simulink model "MPC_backend_main"  (R2026a)
settings: Solver=FixedStepAuto
undefined symbols (not defined in the file or in its folder): acados_nominal_input
libraries: simulink x1
settings Model: Creator=rayyu  LastModifiedBy=rayyu
settings RTWCC: SystemTargetFile=ert.tlc  Description=Embedded Coder
settings ERTTargetCC: GenerateSampleERTMain=on

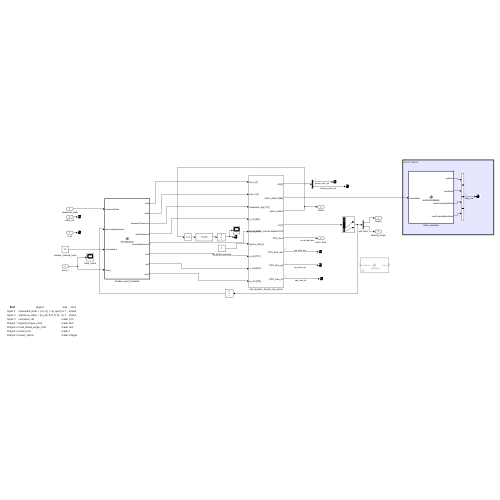
[thumbnail: Simulink's stored preview of the top-level diagram]
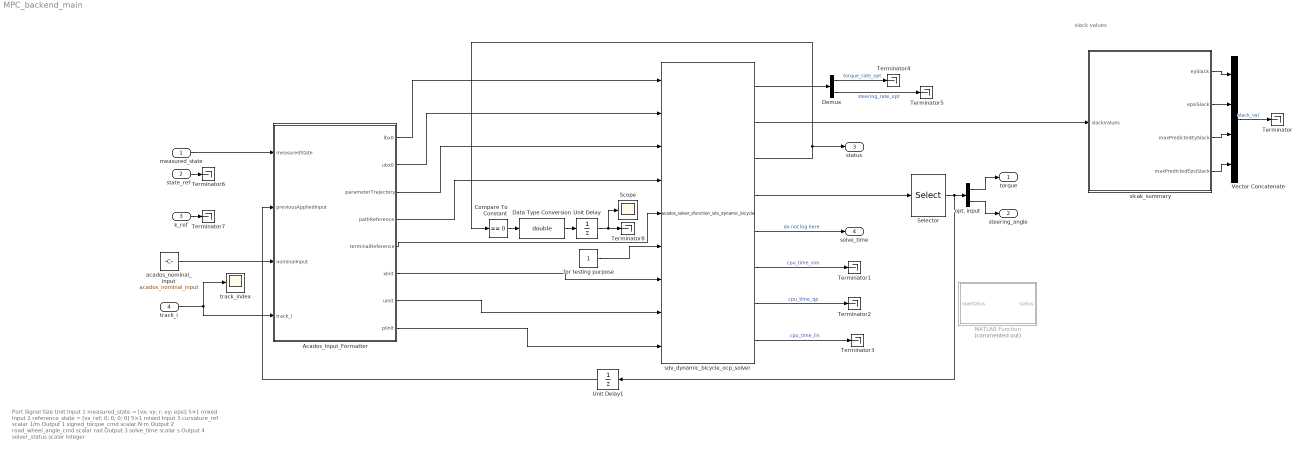
== system MPC_backend_main ==
  note: slack values
  note: Port
      | Signal
      | Size
      | Unit
      |
      | Input 1
      | measured_state = [vx; vy; r; ey; epsi]
      | 5×1
      | mixed
      |
      | Input 2
      | reference_state = [vx_ref; 0; 0; 0; 0]
      | 5×1
      | mixed
      |
      | Input 3
      | curvature_ref
      | scalar
      | 1/m
      |
      | Output 1
      | signed_torque_cmd
      | scalar
      | N·m
      |
      | Output 2
      | road_wheel_angle_cmd
      | scalar
      | rad
      |
      | Output 3
      | solve_time
      | scalar
      | s
      |
      | Output 4
      | solver_status
      | scalar
      | integer
  measured_state : Inport  PortDimensions=[5 1]
  state_ref : Inport  Port=2  PortDimensions=[1 5]
  k_ref : Inport  Port=3  PortDimensions=1
  track_i : Inport  Port=4
  Acados_Input_Formatter : MATLAB Function  TreatAsAtomicUnit=on
  Compare To Constant : simulink/Logic and Bit Operations/Compare To Constant  relop===  const=0  OutDataTypeStr=boolean
  Data Type Conversion : DataTypeConversion  OutDataTypeStr=double  SaturateOnIntegerOverflow=off  RndMeth=Floor
  Demux : Demux  Outputs=2
  MATLAB Function : MATLAB Function  Commented=on  TreatAsAtomicUnit=on
  Scope : Scope
      settings: ActiveDisplayYMinimum=-0.21951243413364641  ActiveDisplayYMaximum=1.6696874989313319
  Selector : Selector  InputPortWidth=7  IndexOptions=Index vector (dialog)  Indices=[6,7]  OutputSizes=1
  Terminator{,1..8} (9 alike) : Terminator
  Unit Delay : UnitDelay  InitialCondition=1  SampleTime=-1
  Unit Delay1 : UnitDelay  SampleTime=-1
  Vector Concatenate : Concatenate  NumInputs=4
  acados_nominal_input : Constant  Value=acados_nominal_input  VectorParams1D=off
  for testing purpose : Constant
  opt. input : Demux  Outputs=2
  sdv_dynamic_bicycle_ocp_solver : S-Function  FunctionName=acados_solver_sfunction_sdv_dynamic_bicycle  SFunctionDeploymentMode=off  EnableBusSupport=off
      mask Display:
      | port_label('input', 1, 'lbx_0 [7]')
      | port_label('input', 2, 'ubx_0 [7]')
      | port_label('input', 3, 'parameter_traj [101]')
      | port_label('input', 4, 'y_ref [891]')
      | port_label('input', 5, 'y_ref_e [5]')
      | port_label('input', 6, 'ignore_inits [1]')
      | port_label('input', 7, 'x_init [707]')
      | port_label('input', 8, 'u_init [200]')
      | port_label('input', 9, 'pi_init [700]')
      | port_label('output', 1, 'u0 [2]')
      | port_label('output', 2, 'slack_values [396]')
      | port_label('output', 3, 'solver_status')
      | port_label('output', 4, 'x1 [7]')
      | port_label('output', 5, 'CPU_time')
      | port_label('output', 6, 'CPU_time_sim')
      | port_label('output', 7, 'CPU_time_qp')
      | port_label('output', 8, 'CPU_time_lin')
      | disp('sdv_dynamic_bicycle acados OCP')
  slcak_summary : MATLAB Function  TreatAsAtomicUnit=on
  track_index : Scope
      settings: ActiveDisplayYMinimum=127.93419653260979  ActiveDisplayYMaximum=131.89125671947426
  torque : Outport
  steering_angle : Outport  Port=2
  status : Outport  Port=3
  solve_time : Outport  Port=4
  wires:
  sdv_dynamic_bicycle_ocp_solver/7 -> Terminator2/1  "cpu_time_qp"
  slcak_summary/3(maxPredictedEySlack) -> Vector Concatenate/3
  opt. input/1 -> torque/1
  Compare To Constant/1 -> Data Type Conversion/1
  Acados_Input_Formatter/5(terminalReference) -> sdv_dynamic_bicycle_ocp_solver/5
  Acados_Input_Formatter/7(uInit) -> sdv_dynamic_bicycle_ocp_solver/8
  Acados_Input_Formatter/2(ubx0) -> sdv_dynamic_bicycle_ocp_solver/2
  measured_state/1 -> Acados_Input_Formatter/1(measuredState)
  track_i/1 -> track_index/1, Acados_Input_Formatter/4(track_i)
  slcak_summary/4(maxPredictedEpsiSlack) -> Vector Concatenate/4
  sdv_dynamic_bicycle_ocp_solver/3 -> Compare To Constant/1, status/1
  sdv_dynamic_bicycle_ocp_solver/1 -> Demux/1
  sdv_dynamic_bicycle_ocp_solver/8 -> Terminator3/1  "cpu_time_lin"
  slcak_summary/2(epsiSlack) -> Vector Concatenate/2
  Vector Concatenate/1 -> Terminator/1  "slack_val"
  sdv_dynamic_bicycle_ocp_solver/5 -> solve_time/1  "do not log here"
  Acados_Input_Formatter/3(parameterTrajectory) -> sdv_dynamic_bicycle_ocp_solver/3
  sdv_dynamic_bicycle_ocp_solver/6 -> Terminator1/1  "cpu_time_sim"
  Data Type Conversion/1 -> Unit Delay/1
  Acados_Input_Formatter/1(lbx0) -> sdv_dynamic_bicycle_ocp_solver/1
  Acados_Input_Formatter/6(xInit) -> sdv_dynamic_bicycle_ocp_solver/7
  acados_nominal_input/1 -> Acados_Input_Formatter/3(nominalInput)
  Acados_Input_Formatter/8(piInit) -> sdv_dynamic_bicycle_ocp_solver/9
  slcak_summary/1(eySlack) -> Vector Concatenate/1
  Acados_Input_Formatter/4(pathReference) -> sdv_dynamic_bicycle_ocp_solver/4
  opt. input/2 -> steering_angle/1
  sdv_dynamic_bicycle_ocp_solver/4 -> Selector/1
  Unit Delay1/1 -> Acados_Input_Formatter/2(previousAppliedInput)
  Selector/1 -> Unit Delay1/1, opt. input/1
  Demux/1 -> Terminator4/1  "torque_rate_opt"
  Demux/2 -> Terminator5/1  "steering_rate_opt"
  Unit Delay/1 -> Terminator8/1, Scope/1
  state_ref/1 -> Terminator6/1
  k_ref/1 -> Terminator7/1
  for testing purpose/1 -> sdv_dynamic_bicycle_ocp_solver/6
  sdv_dynamic_bicycle_ocp_solver/2 -> slcak_summary/1(slackValues)

== matlab function MPC_backend_main/MATLAB Function ==
  data: rawStatus input; status output
function status = mapStatus(rawStatus)
if rawStatus == 0
    status = 1;
else
    status = -1;
end

end

== matlab function MPC_backend_main/Acados_Input_Formatter ==
  data: measuredState input; previousAppliedInput input; nominalInput input; track_i input; track_ref_table parameter; lbx0 output; ubx0 output; parameterTrajectory output; pathReference output; terminalReference output; xInit output; uInit output; piInit output
function [ ...
    lbx0, ...
    ubx0, ...
    parameterTrajectory, ...
    pathReference, ...
    terminalReference, ...
    xInit, ...
    uInit, ...
    piInit] = ...
    formatInputs( ...
        measuredState, ...
        previousAppliedInput, ...
        nominalInput, ... % only for tracking the input
        track_i, ...
        track_ref_table)

numberOfIntervals = 100;
predictionStep_s = 0.01;

numberOfStates = 7;
numberOfInputs = 2;
numberOfCostOutputs = 9;

%% Current augmented state
%
% measuredState:
%   [vx; vy; r; ey; epsi]
%
% previousAppliedInput:
%   [frontAxleTorque; roadWheelAngle]

augmentedMeasuredState = [
    measuredState
    previousAppliedInput
    ];

%% Preallocate fixed-size outputs

lbx0 = zeros(7,1);
ubx0 = zeros(7,1);

parameterTrajectory = zeros(numberOfIntervals + 1,1);
pathReference = zeros(numberOfCostOutputs * (numberOfIntervals - 1),1); % numberofinterval * numberofoutputs - numberofoutputs

xInitRows = (numberOfIntervals + 1) * numberOfStates;
uInitRows = numberOfInputs * numberOfIntervals;
piInitRows = numberOfStates * numberOfIntervals;
xInit = zeros(xInitRows,1); % (numberOfInterval + 1) * numberOfStates 
uInit = zeros(uInitRows,1);
piInit = zeros(piInitRows,1);

%% Preview indices for nodes 0 through N

numberOfTrackPoints = size(track_ref_table,1);
previewIndices = ones(numberOfIntervals + 1,1);

currentIndex = round(track_i); 
currentIndex = max( ...
    1, min(currentIndex, numberOfTrackPoints));

previewIndices(1) = currentIndex;

minimumPreviewSpeed_mps = 1;

predictedStation_m = ...
    track_ref_table(currentIndex,1);

for node = 2:(numberOfIntervals + 1)

    currentIndex = previewIndices(node - 1);

    predictedSpeed_mps = max( ...
        track_ref_table(currentIndex, 6), ...
        minimumPreviewSpeed_mps);

    predictedStation_m = ...
        predictedStation_m ...
        + predictedSpeed_mps*predictionStep_s;

    nextIndex = currentIndex;

    while nextIndex < numberOfTrackPoints && ...
            track_ref_table(nextIndex,1) ...
            < predictedStation_m

        nextIndex = nextIndex + 1;
    end

    previewIndices(node) = nextIndex;
end

%% Curvature preview: nodes 0 through N

for node = 1:(numberOfIntervals + 1)

    referenceIndex = previewIndices(node);

    parameterTrajectory(node) = ...
        track_ref_table(referenceIndex,5);
end

%% References for stages 1 through N-1
%
% Stage cost output:
% [vx; vy; r; ey; epsi; torque; steering; torqueRate; steeringRate]

for stage = 1:(numberOfIntervals - 1)

    referenceIndex = previewIndices(stage + 1);

    speedReference_mps = ...
        track_ref_table(referenceIndex,6);

    yawRateReference_radps = ...
        track_ref_table(referenceIndex,7);

    stageReference = [
        speedReference_mps
        0
        yawRateReference_radps
        0
        0
        0
        0
        0
        0
        ];

    outputStartIndex = ...
        (stage - 1)*numberOfCostOutputs + 1;

    for element = 1:numberOfCostOutputs
        pathReference( ...
            outputStartIndex + element - 1) = ...
            stageReference(element);
    end
end

%% Fix augmented state at prediction node zero

for stateIndex = 1:numberOfStates

    lbx0(stateIndex) = ...
        augmentedMeasuredState(stateIndex);

    ubx0(stateIndex) = ...
        augmentedMeasuredState(stateIndex);
end

%% Terminal reference at node N

terminalIndex = ...
    previewIndices(numberOfIntervals + 1);

terminalReference = [
    track_ref_table(terminalIndex,6)
    0
    track_ref_table(terminalIndex,7)
    0
    0
    ];

%% External state-trajectory initialization

for stage = 0:numberOfIntervals

    startIndex = stage*numberOfStates + 1;

    for stateIndex = 1:numberOfStates

        xInit(startIndex + stateIndex - 1) = ...
            augmentedMeasuredState(stateIndex);
    end
end

%% External rate-input initialization
%
% The optimizer inputs are torque rate and steering rate.
% Their nominal values are zero—not nominal torque and steering.

for stage = 0:(numberOfIntervals - 1)

    startIndex = stage*numberOfInputs + 1;

    uInit(startIndex) = 0;
    uInit(startIndex + 1) = 0;
end

end

== matlab function MPC_backend_main/slcak_summary ==
  data: slackValues input; eySlack output; epsiSlack output; maxPredictedEySlack output; maxPredictedEpsiSlack output
function [eySlack, epsiSlack, ...
          maxPredictedEySlack, ...
          maxPredictedEpsiSlack] = ...
          summarizeSlacks(slackValues)

% Two states, each having lower and upper slack.
slackByStage = reshape(slackValues, 4, []);

lowerEy   = slackByStage(1,:);
lowerEpsi = slackByStage(2,:);
upperEy   = slackByStage(3,:);
upperEpsi = slackByStage(4,:);

% Violation predicted at the first constrained prediction stage.
eySlack = max(lowerEy(1), upperEy(1));
epsiSlack = max(lowerEpsi(1), upperEpsi(1));

% Largest violation anywhere in the current prediction horizon.
maxPredictedEySlack = ...
    max(max(lowerEy, upperEy));

maxPredictedEpsiSlack = ...
    max(max(lowerEpsi, upperEpsi));

end
